simulink model "Prob_5"  (R2016a)
settings: Solver=VariableStepAuto  StartTime=0.0  StopTime=10.0  RelTol=1e-3
values from neighbouring files (symbols this model uses):
  C = 1e-05    [MAT_file.mat]
  R = 10    [MAT_file.mat]
libraries: simulink x1
settings Model: Creator=Admin  LastModifiedBy=Admin

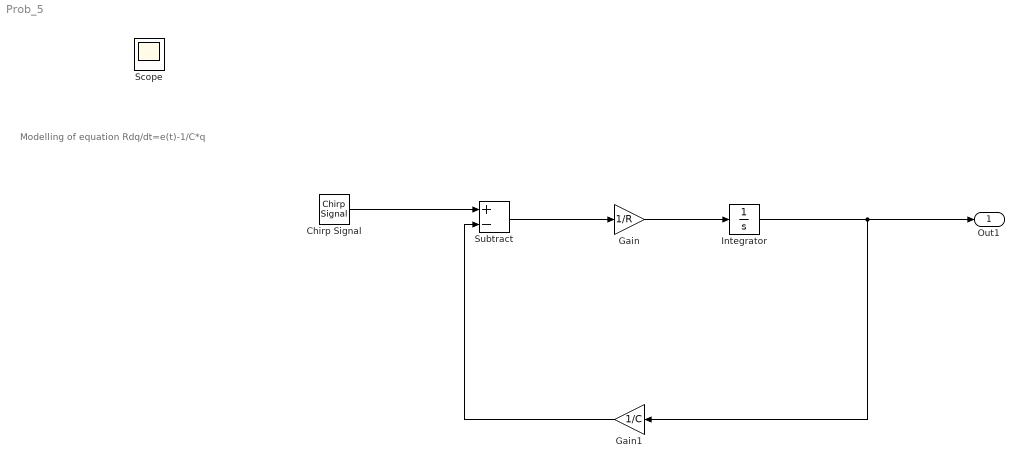
== system Prob_5 ==
  note: Modelling of equation
      | Rdq/dt=e(t)-1/C*q
  Chirp Signal : simulink/Sources/Chirp Signal  f1=0.1  T=100  f2=1
  Gain : Gain  Gain=1/R
  Gain1 : Gain  Gain=1/C
  Integrator : Integrator
  Subtract : Sum  Inputs=+-
  Out1 : Outport
  Scope : Scope
  wires:
  Chirp Signal/1 -> Subtract/1
  Gain/1 -> Integrator/1
  Integrator/1 -> Gain1/1, Out1/1
  Subtract/1 -> Gain/1
  Gain1/1 -> Subtract/2
